simulink model "es3sim"  (R2023b)
settings: Solver=VariableStepAuto  StartTime=0.0  StopTime=Tfin  RelTol=1e-3
values from neighbouring files (symbols this model uses):
  beta0 = [0 0 0]'    [es2.m]    (also in es3.m)
  IJ = inv(J)    [es1.m]    (also in es2.m; es3.m)
  J = [937.5 833.3 270.8]    [dyn_kin_quat.m]    (also in es1.m = diag([937.5, 833.3, 270.8]); es2.m = diag([937.5, 833.3, 270.8]); es3.m = diag([937.5, 833.3, 270.8]); euler_eq.m = [400 50 150])
  M = [0,0,0]'    [es1.m]    (also in es2.m = [0 0 0]; es3.m = [0 0 0])
  w0 = [1,0.1,0]'    [es1.m]    (also in es2.m; es3.m)
libraries: vrlib x1
settings Model: Creator=luigi  LastModifiedBy=luigi

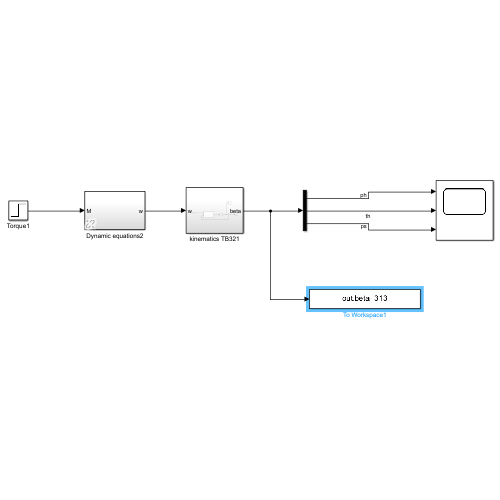
[thumbnail: Simulink's stored preview of the top-level diagram]
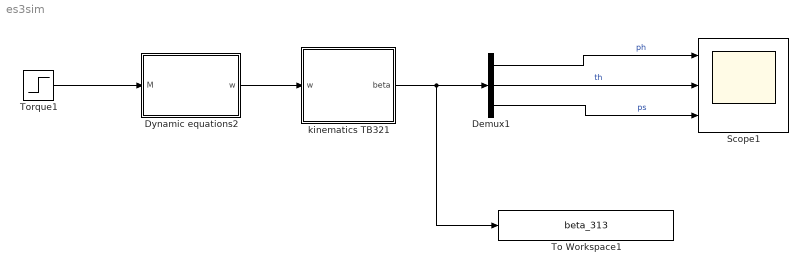
== system es3sim ==
  Demux1 : Demux  Outputs=3
  Dynamic equations2 : Subsystem  AncestorBlock=lib_rotations_2014/Euler equation
  Scope1 : Scope  NumInputPorts=3
  To Workspace1 : ToWorkspace  VariableName=beta_313  SaveFormat=Timeseries  SampleTime=-1
  Torque1 : Step  Time=0  After=M  SampleTime=0
  kinematics TB321 : Subsystem
  wires:
  Demux1/1 -> Scope1/1  "ph"
  Demux1/3 -> Scope1/3  "ps"
  Torque1/1 -> Dynamic equations2/1(M)
  kinematics TB321/1(beta) -> Demux1/1, To Workspace1/1
  Demux1/2 -> Scope1/2  "th"
  Dynamic equations2/1(w) -> kinematics TB321/1(w)

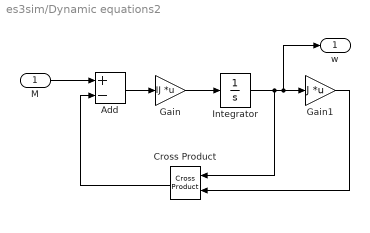
== system es3sim/Dynamic equations2 ==
  M : Inport
  Add : Sum  Inputs=+-
  Cross Product : vrlib/Utilities/Cross Product
  Gain : Gain  Gain=IJ  Multiplication=Matrix(K*u)
  Gain1 : Gain  Gain=J  Multiplication=Matrix(K*u)
  Integrator : Integrator  InitialCondition=w0
  w : Outport  VectorParamsAs1DForOutWhenUnconnected=off
  wires:
  Cross Product/1 -> Add/2
  Add/1 -> Gain/1
  Gain1/1 -> Cross Product/2
  Gain/1 -> Integrator/1
  Integrator/1 -> Gain1/1, w/1, Cross Product/1
  M/1 -> Add/1

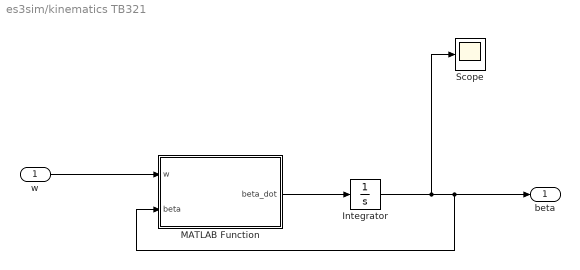
== system es3sim/kinematics TB321 ==
  w : Inport  PortDimensions=3
  Integrator : Integrator  InitialCondition=beta0
  MATLAB Function : MATLAB Function  TreatAsAtomicUnit=on
  Scope : Scope
  beta : Outport  PortDimensions=3  VectorParamsAs1DForOutWhenUnconnected=off
  wires:
  w/1 -> MATLAB Function/1(w)
  MATLAB Function/1(beta_dot) -> Integrator/1
  Integrator/1 -> beta/1, MATLAB Function/2(beta), Scope/1

== matlab function es3sim/kinematics TB321/MATLAB Function ==
  data: w input; beta_dot output; beta input
function beta_dot = kinTB_313(w,beta)
%The function kinTB_313(w,beta) compute the kinematics of TB-313 using the
%inverse of the DCM matrix. The parametres are omega, the angular velocity,
%and angles.

phi = beta(1);
theta = beta(2);
psi = beta(3);

T = [sin(psi) cos(psi) 0
    sin(theta)*cos(psi) -sin(theta)*sin(psi) 0
    -cos(theta)*sin(psi) -cos(theta)*cos(psi) sin(theta)];
T = 1*T;

beta_dot = T*w;
end
